simulink model "final_model"  (R2021b)
settings: Solver=VariableStepAuto  StartTime=0.0  StopTime=10  RelTol=1e-3
libraries: spsMeanLib x9, spsDiodeLib x7, spsSeriesRLCBranchLib x5, spsACVoltageSourceLib x3, spsVoltageMeasurementLib x3, spsCurrentMeasurementLib x2, spsDCMachineLib x1, spsDCVoltageSourceLib x1, spsMosfetLib x1, spsPWMGeneratorDCDCLib x1, eePowerMeasurement x1, spspowerguiLib x1
settings Model: Creator=pc  LastModifiedBy=Emre Çakmakyurdu
settings SolverCC: ZeroCrossAlgorithm=Adaptive
settings DebuggingCC: IgnoredZcDiagnostic=none

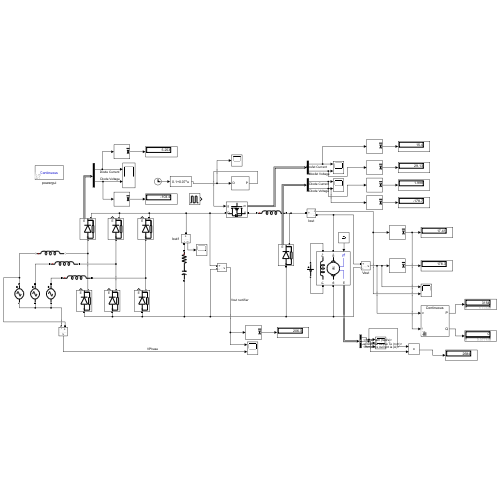
[thumbnail: Simulink's stored preview of the top-level diagram]
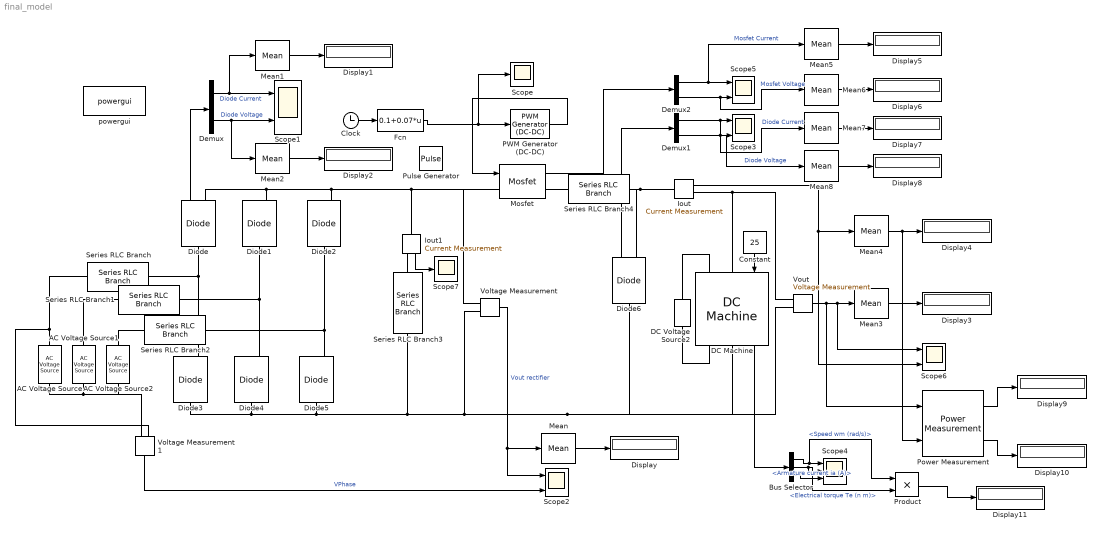
== system final_model ==
  AC Voltage Source : spsACVoltageSourceLib/AC Voltage Source  Amplitude=90*sqrt(2)  Phase=0  Frequency=50  SampleTime=0  Measurements=None  BusType=swing  Pref=10e3  Qref=0  Qmin=-inf  Qmax=+inf
  AC Voltage Source1 : spsACVoltageSourceLib/AC Voltage Source  Amplitude=90*sqrt(2)  Phase=-120  Frequency=50  SampleTime=0  Measurements=None  BusType=swing  Pref=10e3  Qref=0  Qmin=-inf  Qmax=+inf
  AC Voltage Source2 : spsACVoltageSourceLib/AC Voltage Source  Amplitude=90*sqrt(2)  Phase=120  Frequency=50  SampleTime=0  Measurements=None  BusType=swing  Pref=10e3  Qref=0  Qmin=-inf  Qmax=+inf
  Bus Selector : BusSelector  OutputSignals=Speed wm (rad/s),Electrical torque Te (n m),Armature current ia (A)
  Clock : Clock
  Constant : Constant  Value=25
  DC Machine : spsDCMachineLib/DC Machine  PresetModel=No  MechanicalLoad=Torque TL  FieldType=Wound  ShowDetailedParameters=on  MeasurementBus=off  RLa="[ 1.07  0.0245]"  RLf="[ 210  23]"  Laf=1.8  MachineConstant=Torque constant (N.m/A)  Ke=1.8  Kt=1.8  J=1  Bm=0  Tf=0  w0=1  Ifinit=1.04761904756944  TsPowergui=0  TsBlock=-1
  DC Voltage Source2 : spsDCVoltageSourceLib/DC Voltage Source  Amplitude=220  Measurements=None
  Demux : Demux  Outputs=2
  Demux1 : Demux  Outputs=2
  Demux2 : Demux  Outputs=2
  Diode{,1..6} (7 alike) : spsDiodeLib/Diode  Ron=0.001  Lon=0  Vf=0.8  IC=0  UseSnubber=0  Rs=500  Cs=250e-9  Measurements=on
  Display{,1..11} (12 alike) : Display
  Fcn : Fcn  Expr=0.1+0.07*u
  Iout : spsCurrentMeasurementLib/Current Measurement  PhasorSimulation=off  OutputType=Complex  PSBequivalent=0
  Iout1 : spsCurrentMeasurementLib/Current Measurement  PhasorSimulation=off  OutputType=Complex  PSBequivalent=0
  Mean{,1..8} (9 alike) : spsMeanLib/Mean  Freq=50  Vinit=0  Ts=0
  Mosfet : spsMosfetLib/Mosfet  Ron=0.1  Lon=0  Rd=0.01  Vfd=0.7  IC=0  Rs=500  Cs=250e-9  Measurements=on
  PWM Generator (DC-DC) : spsPWMGeneratorDCDCLib/PWM Generator (DC-DC)  Fsw=1000  Ts=0
  Power Measurement : eePowerMeasurement/Power Measurement  LabelModeActiveChoice=Continuous  F=50  K=[0 1 2 3]  Ts=0
      settings: SourceProductBaseCode=PS
  Product : Product
  Pulse Generator : DiscretePulseGenerator  PulseType=Time based  Period=1/10000  PulseWidth=80
  Scope : Scope
  Scope{1..3,5..6} (5 alike) : Scope  NumInputPorts=2
  Scope4 : Scope  NumInputPorts=3
  Scope7 : Scope
  Series RLC Branch{,1..2,4} (4 alike) : spsSeriesRLCBranchLib/Series RLC Branch  LConnTagsString=__new0  RConnTagsString=__new0  BranchType=L  Resistance=1  Inductance=0.5e-3  SetiL0=off  InitialCurrent=0  Capacitance=1e-6  Setx0=off  InitialVoltage=0  Measurements=None
  Series RLC Branch3 : spsSeriesRLCBranchLib/Series RLC Branch  LConnTagsString=__new0  RConnTagsString=__new0  BranchType=RC  Resistance=0.0001  Inductance=1e-3  SetiL0=off  InitialCurrent=0  Capacitance=100e-6  Setx0=off  InitialVoltage=0  Measurements=None
  Voltage Measurement : spsVoltageMeasurementLib/Voltage Measurement  PhasorSimulation=off  OutputType=Complex  PSBequivalent=0
  Voltage Measurement1 : spsVoltageMeasurementLib/Voltage Measurement  PhasorSimulation=off  OutputType=Complex  PSBequivalent=0
  Vout : spsVoltageMeasurementLib/Voltage Measurement  PhasorSimulation=off  OutputType=Complex  PSBequivalent=0
  powergui : spspowerguiLib/powergui  Priority=1  SimulationMode=Continuous  SampleTime=50e-6  frequency=60  Iterations=50  frequencyindice=0  Pbase=100e6  ErrMax=1e-4  UnitsV=kV  UnitsW=MW  buscounter=0  FunctionMessages=off  echomessages=off  EnableUseOfTLC=off  CurrentSourceSwitches=off  DisableSnubberDevices=off  DisableRonSwitches=off  DisableVfSwitches=off  DisplayEquations=off  AutomaticDiscreteSolvers=off  SolverType=Tustin/Backward Euler (TBE)  Interpol=off  ExternalGateDelay=off  methode=off  Ts=100  x0status=blocks  SPID=on  SwTol=0  HookPort=off  NonlinearTolerance=1e-4  nMaxIteration=100  ContinueOnMaxIteration=off  RestoreLinks=warning  ResistiveCurrentMeasurement=off  Frange=[0:2:500]  Ylog=off  Xlog=on  ShowGrid=off  save=off  variable=ZData  structure=0  ZoomFFT=off  StartTime=0.0  cycles=1  DisplayStyle=1  fundamental=60  FreqAxis=off  MaxFrequency=1000  frequencyindicesteady=1  RmsSteady=1  display=off
  wires:
  Demux/1 -> Mean1/1, Scope1/1  "Diode Current"
  Power Measurement/2 -> Display10/1
  Power Measurement/1 -> Display9/1
  Constant/1 -> DC Machine/1
  Clock/1 -> Fcn/1
  Mean8/1 -> Display8/1
  Mosfet/1 -> Demux2/1
  Iout/1 -> Scope6/2, Mean4/1
  Voltage Measurement1/1 -> Scope2/2  "VPhase"
  Mean5/1 -> Display5/1
  Mean7/1 -> Display7/1
  Mean4/1 -> Power Measurement/2, Display4/1
  Mean6/1 -> Display6/1
  Diode6/1 -> Demux1/1
  Mean3/1 -> Display3/1
  Demux1/2 -> Mean8/1, Scope3/2  "Diode Voltage"
  Demux1/1 -> Mean7/1, Scope3/1  "Diode Current"
  Diode/1 -> Demux/1
  Mean/1 -> Display/1
  Voltage Measurement/1 -> Scope2/1, Mean/1  "Vout rectifier"
  Demux2/2 -> Mean6/1, Scope5/2  "Mosfet Voltage"
  Vout/1 -> Power Measurement/1, Scope6/1, Mean3/1
  Demux/2 -> Mean2/1, Scope1/2  "Diode Voltage"
  Mean1/1 -> Display1/1
  Demux2/1 -> Mean5/1, Scope5/1  "Mosfet Current"
  Iout1/1 -> Scope7/1
  Mean2/1 -> Display2/1
  DC Machine/1 -> Bus Selector/1
  Bus Selector/1 -> Product/1, Scope4/1  "<Speed wm (rad/s)>"
  Bus Selector/2 -> Product/2, Scope4/2  "<Electrical torque Te (n m)>"
  Bus Selector/3 -> Scope4/3  "<Armature current ia (A)>"
  Product/1 -> Display11/1
  PWM Generator (DC-DC)/1 -> Mosfet/1
  Fcn/1 -> Scope/1, PWM Generator (DC-DC)/1
  connections:
  Diode4/LConn1 -- Diode3/LConn1 -- Diode5/LConn1 -- Series RLC Branch3/RConn1 -- Voltage Measurement/LConn2 -- Vout/LConn2 -- DC Machine/RConn1 -- Diode6/LConn1
  DC Machine/LConn1 -- Iout/RConn1 -- Vout/LConn1
  Iout1/LConn1 -- Diode/RConn1 -- Diode1/RConn1 -- Diode2/RConn1 -- Voltage Measurement/LConn1 -- Mosfet/LConn1
  AC Voltage Source1/LConn1 -- AC Voltage Source/LConn1 -- Voltage Measurement1/LConn2 -- AC Voltage Source2/LConn1
  Diode1/LConn1 -- Series RLC Branch1/RConn1 -- Diode4/RConn1
  Diode2/LConn1 -- Diode5/RConn1 -- Series RLC Branch2/RConn1
  Diode/LConn1 -- Series RLC Branch/RConn1 -- Diode3/RConn1
  Diode6/RConn1 -- Series RLC Branch4/RConn1 -- Iout/LConn1
  Series RLC Branch3/LConn1 -- Iout1/RConn1
  DC Machine/LConn2 -- DC Voltage Source2/RConn1
  DC Machine/RConn2 -- DC Voltage Source2/LConn1
  Voltage Measurement1/LConn1 -- Series RLC Branch/LConn1 -- AC Voltage Source/RConn1
  AC Voltage Source1/RConn1 -- Series RLC Branch1/LConn1
  AC Voltage Source2/RConn1 -- Series RLC Branch2/LConn1
  Mosfet/RConn1 -- Series RLC Branch4/LConn1
